simulink library "halin"  (R2021b)
settings: Solver=VariableStepAuto  StartTime=0.0  StopTime=10.0  RelTol=1e-3
undefined symbols (not defined in the file): KHAL_CAN1ABM1E2E_flg, KHAL_CAN1EPB1E2E_flg, KHAL_CAN1EPS1E2E_flg, KHAL_CAN1ESC1E2E_flg, KHAL_CAN1ESC5E2E_flg, KHAL_CAN3BMS1E2E_flg, KHAL_CAN3BMS6E2E_flg, KHAL_CAN3CCU1E2E_flg, KHAL_CAN3CCU2E2E_flg, KHAL_CAN3MCUNF1E2E_flg, KHAL_CAN3MCUNR1E2E_flg, KHAL_CAN3Shifter1E2E_flg, KHAL_CAN3Shifter2E2E_flg, KHAL_CAN6FCM2E2E_flg, KHAL_CAN6FCM4E2E_flg, TRUE
libraries: simulink x645, FVT_lib x207, hcu_lib x59
(part 16 of 23)

== system halin/HAL_IN/CAN4/zGW_LINFr2 ==
  DT_CAN4_SG_zGW_LINFr2 : Inport
  EWP1BlockError : Subsystem
  EWP1OverCurrError : Subsystem
  EWP2BlockError : Subsystem
  EWP2OverCurrError : Subsystem
  EWP3BlockError : Subsystem
  EWP3OverCurrError : Subsystem
  bus_selector : BusSelector  OutputSignals=CAN4_EWP1_Block_Error
  bus_selector1 : BusSelector  OutputSignals=CAN4_EWP1_OverCurr_Error
  bus_selector2 : BusSelector  OutputSignals=CAN4_EWP2_Block_Error
  bus_selector3 : BusSelector  OutputSignals=CAN4_EWP2_OverCurr_Error
  bus_selector4 : BusSelector  OutputSignals=CAN4_EWP3_Block_Error
  bus_selector5 : BusSelector  OutputSignals=CAN4_EWP3_OverCurr_Error
  VHAL_EWP1BlockError_enum : Outport
  VHAL_EWP1OverCurrError_enum : Outport  Port=2
  VHAL_EWP2BlockError_enum : Outport  Port=3
  VHAL_EWP2OverCurrError_enum : Outport  Port=4
  VHAL_EWP3BlockError_enum : Outport  Port=5
  VHAL_EWP3OverCurrError_enum : Outport  Port=6
  wires:
  DT_CAN4_SG_zGW_LINFr2/1 -> [DT_CAN4_SG_zGW_LINFr2]
  [DT_CAN4_SG_zGW_LINFr2] -> bus_selector/1
  bus_selector/1 -> EWP1BlockError/1(EWP1_Block_Error)  "<CAN4_EWP1_Block_Error>"
  EWP1BlockError/1(VHAL_EWP1BlockError_enum) -> VHAL_EWP1BlockError_enum/1
  [DT_CAN4_SG_zGW_LINFr2] -> bus_selector1/1
  bus_selector1/1 -> EWP1OverCurrError/1(EWP1_OverCurr_Error)  "<CAN4_EWP1_OverCurr_Error>"
  EWP1OverCurrError/1(VHAL_EWP1OverCurrError_enum) -> VHAL_EWP1OverCurrError_enum/1
  [DT_CAN4_SG_zGW_LINFr2] -> bus_selector2/1
  bus_selector2/1 -> EWP2BlockError/1(EWP2_Block_Error)  "<CAN4_EWP2_Block_Error>"
  EWP2BlockError/1(VHAL_EWP2BlockError_enum) -> VHAL_EWP2BlockError_enum/1
  [DT_CAN4_SG_zGW_LINFr2] -> bus_selector3/1
  bus_selector3/1 -> EWP2OverCurrError/1(EWP2_OverCurr_Error)  "<CAN4_EWP2_OverCurr_Error>"
  EWP2OverCurrError/1(VHAL_EWP2OverCurrError_enum) -> VHAL_EWP2OverCurrError_enum/1
  [DT_CAN4_SG_zGW_LINFr2] -> bus_selector4/1
  bus_selector4/1 -> EWP3BlockError/1(EWP3_Block_Error)  "<CAN4_EWP3_Block_Error>"
  EWP3BlockError/1(VHAL_EWP3BlockError_enum) -> VHAL_EWP3BlockError_enum/1
  [DT_CAN4_SG_zGW_LINFr2] -> bus_selector5/1
  bus_selector5/1 -> EWP3OverCurrError/1(EWP3_OverCurr_Error)  "<CAN4_EWP3_OverCurr_Error>"
  EWP3OverCurrError/1(VHAL_EWP3OverCurrError_enum) -> VHAL_EWP3OverCurrError_enum/1

== system halin/HAL_IN/CAN4/zGW_SEAT1 ==
  DT_CAN4_SG_zGW_SEAT1 : Inport
  DSEATAntiSta : Subsystem
  DSEATEntryFunSta : Subsystem
  DSEATErrorSta : Subsystem
  DSEATHWVer : Subsystem
  DSEATMode : Subsystem
  DSEATSWVer : Subsystem
  DSEATVentSta : Subsystem
  DSEATheatersta : Subsystem
  PSEATErrorSta : Subsystem
  PSEATHWVer : Subsystem
  PSEATMode : Subsystem
  PSEATSWVer : Subsystem
  PSEATVentSta : Subsystem
  PSEATheatersta : Subsystem
  bus_selector : BusSelector  OutputSignals=CAN4_DSEAT_Anti_Sta
  bus_selector1 : BusSelector  OutputSignals=CAN4_DSEAT_EntryFun_Sta
  bus_selector10 : BusSelector  OutputSignals=CAN4_PSEAT_Mode
  bus_selector11 : BusSelector  OutputSignals=CAN4_PSEAT_SW_Ver
  bus_selector12 : BusSelector  OutputSignals=CAN4_PSEAT_Vent_Sta
  bus_selector13 : BusSelector  OutputSignals=CAN4_PSEAT_heater_sta
  bus_selector2 : BusSelector  OutputSignals=CAN4_DSEAT_Error_Sta
  bus_selector3 : BusSelector  OutputSignals=CAN4_DSEAT_HW_Ver
  bus_selector4 : BusSelector  OutputSignals=CAN4_DSEAT_Mode
  bus_selector5 : BusSelector  OutputSignals=CAN4_DSEAT_SW_Ver
  bus_selector6 : BusSelector  OutputSignals=CAN4_DSEAT_Vent_Sta
  bus_selector7 : BusSelector  OutputSignals=CAN4_DSEAT_heater_sta
  bus_selector8 : BusSelector  OutputSignals=CAN4_PSEAT_Error_Sta
  bus_selector9 : BusSelector  OutputSignals=CAN4_PSEAT_HW_Ver
  VHAL_DSEATAntiSta_flg : Outport
  VHAL_DSEATEntryFunSta_flg : Outport  Port=2
  VHAL_DSEATErrorSta_flg : Outport  Port=3
  VHAL_DSEATHWVer_enum : Outport  Port=4
  VHAL_DSEATMode_enum : Outport  Port=5
  VHAL_DSEATSWVer_enum : Outport  Port=6
  VHAL_DSEATVentSta_enum : Outport  Port=7
  VHAL_DSEATheatersta_enum : Outport  Port=8
  VHAL_PSEATErrorSta_flg : Outport  Port=9
  VHAL_PSEATHWVer_enum : Outport  Port=10
  VHAL_PSEATMode_enum : Outport  Port=11
  VHAL_PSEATSWVer_enum : Outport  Port=12
  VHAL_PSEATVentSta_enum : Outport  Port=13
  VHAL_PSEATheatersta_enum : Outport  Port=14
  wires:
  DT_CAN4_SG_zGW_SEAT1/1 -> [DT_CAN4_SG_zGW_SEAT1]
  [DT_CAN4_SG_zGW_SEAT1] -> bus_selector/1
  bus_selector/1 -> DSEATAntiSta/1(DSEAT_Anti_Sta)  "<CAN4_DSEAT_Anti_Sta>"
  DSEATAntiSta/1(VHAL_DSEATAntiSta_flg) -> VHAL_DSEATAntiSta_flg/1
  [DT_CAN4_SG_zGW_SEAT1] -> bus_selector1/1
  bus_selector1/1 -> DSEATEntryFunSta/1(DSEAT_EntryFun_Sta)  "<CAN4_DSEAT_EntryFun_Sta>"
  DSEATEntryFunSta/1(VHAL_DSEATEntryFunSta_flg) -> VHAL_DSEATEntryFunSta_flg/1
  [DT_CAN4_SG_zGW_SEAT1] -> bus_selector2/1
  bus_selector2/1 -> DSEATErrorSta/1(DSEAT_Error_Sta)  "<CAN4_DSEAT_Error_Sta>"
  DSEATErrorSta/1(VHAL_DSEATErrorSta_flg) -> VHAL_DSEATErrorSta_flg/1
  [DT_CAN4_SG_zGW_SEAT1] -> bus_selector3/1
  bus_selector3/1 -> DSEATHWVer/1(DSEAT_HW_Ver)  "<CAN4_DSEAT_HW_Ver>"
  DSEATHWVer/1(VHAL_DSEATHWVer_enum) -> VHAL_DSEATHWVer_enum/1
  [DT_CAN4_SG_zGW_SEAT1] -> bus_selector4/1
  bus_selector4/1 -> DSEATMode/1(DSEAT_Mode)  "<CAN4_DSEAT_Mode>"
  DSEATMode/1(VHAL_DSEATMode_enum) -> VHAL_DSEATMode_enum/1
  [DT_CAN4_SG_zGW_SEAT1] -> bus_selector5/1
  bus_selector5/1 -> DSEATSWVer/1(DSEAT_SW_Ver)  "<CAN4_DSEAT_SW_Ver>"
  DSEATSWVer/1(VHAL_DSEATSWVer_enum) -> VHAL_DSEATSWVer_enum/1
  [DT_CAN4_SG_zGW_SEAT1] -> bus_selector6/1
  bus_selector6/1 -> DSEATVentSta/1(DSEAT_Vent_Sta)  "<CAN4_DSEAT_Vent_Sta>"
  DSEATVentSta/1(VHAL_DSEATVentSta_enum) -> VHAL_DSEATVentSta_enum/1
  [DT_CAN4_SG_zGW_SEAT1] -> bus_selector7/1
  bus_selector7/1 -> DSEATheatersta/1(DSEAT_heater_sta)  "<CAN4_DSEAT_heater_sta>"
  DSEATheatersta/1(VHAL_DSEATheatersta_enum) -> VHAL_DSEATheatersta_enum/1
  [DT_CAN4_SG_zGW_SEAT1] -> bus_selector8/1
  bus_selector8/1 -> PSEATErrorSta/1(PSEAT_Error_Sta)  "<CAN4_PSEAT_Error_Sta>"
  PSEATErrorSta/1(VHAL_PSEATErrorSta_flg) -> VHAL_PSEATErrorSta_flg/1
  [DT_CAN4_SG_zGW_SEAT1] -> bus_selector9/1
  bus_selector9/1 -> PSEATHWVer/1(PSEAT_HW_Ver)  "<CAN4_PSEAT_HW_Ver>"
  PSEATHWVer/1(VHAL_PSEATHWVer_enum) -> VHAL_PSEATHWVer_enum/1
  [DT_CAN4_SG_zGW_SEAT1] -> bus_selector10/1
  bus_selector10/1 -> PSEATMode/1(PSEAT_Mode)  "<CAN4_PSEAT_Mode>"
  PSEATMode/1(VHAL_PSEATMode_enum) -> VHAL_PSEATMode_enum/1
  [DT_CAN4_SG_zGW_SEAT1] -> bus_selector11/1
  bus_selector11/1 -> PSEATSWVer/1(PSEAT_SW_Ver)  "<CAN4_PSEAT_SW_Ver>"
  PSEATSWVer/1(VHAL_PSEATSWVer_enum) -> VHAL_PSEATSWVer_enum/1
  [DT_CAN4_SG_zGW_SEAT1] -> bus_selector12/1
  bus_selector12/1 -> PSEATVentSta/1(PSEAT_Vent_Sta)  "<CAN4_PSEAT_Vent_Sta>"
  PSEATVentSta/1(VHAL_PSEATVentSta_enum) -> VHAL_PSEATVentSta_enum/1
  [DT_CAN4_SG_zGW_SEAT1] -> bus_selector13/1
  bus_selector13/1 -> PSEATheatersta/1(PSEAT_heater_sta)  "<CAN4_PSEAT_heater_sta>"
  PSEATheatersta/1(VHAL_PSEATheatersta_enum) -> VHAL_PSEATheatersta_enum/1

== system halin/HAL_IN/CAN5/VHAL_CANMsgInvalidTBOX1_flg ==
  Cast To Boolean13 : DataTypeConversion  OutDataTypeStr=boolean
  Constant : Constant  Value=TRUE
  Latch13 : hcu_lib/Basic_Blocks/Latch
  Switch13 : Switch  Criteria=u2 ~= 0
  Unit Delay : UnitDelay  SampleTime=-1  HasFrameUpgradeWarning=on
  UnitConverter : DataTypeConversion  OutDataTypeStr=boolean
  Out : Outport
  wires:
  Constant/1 -> Switch13/3
  Unit Delay/1 -> Cast To Boolean13/1
  Cast To Boolean13/1 -> Switch13/1, Latch13/1
  Switch13/1 -> UnitConverter/1
  Latch13/1 -> Switch13/2
  UnitConverter/1 -> Unit Delay/1, Out/1  "VHAL_CANMsgInvalidTBOX1_flg"

== system halin/HAL_IN/CAN5/VHAL_CANMsgInvalidTBOX2_flg ==
  Cast To Boolean13 : DataTypeConversion  OutDataTypeStr=boolean
  Constant : Constant  Value=TRUE
  Latch13 : hcu_lib/Basic_Blocks/Latch
  Switch13 : Switch  Criteria=u2 ~= 0
  Unit Delay : UnitDelay  SampleTime=-1  HasFrameUpgradeWarning=on
  UnitConverter : DataTypeConversion  OutDataTypeStr=boolean
  Out : Outport
  wires:
  Constant/1 -> Switch13/3
  Unit Delay/1 -> Cast To Boolean13/1
  Cast To Boolean13/1 -> Switch13/1, Latch13/1
  Switch13/1 -> UnitConverter/1
  Latch13/1 -> Switch13/2
  UnitConverter/1 -> Unit Delay/1, Out/1  "VHAL_CANMsgInvalidTBOX2_flg"

== system halin/HAL_IN/CAN5/VHAL_CANMsgInvalidTBOX3_flg ==
  Cast To Boolean13 : DataTypeConversion  OutDataTypeStr=boolean
  Constant : Constant  Value=TRUE
  Latch13 : hcu_lib/Basic_Blocks/Latch
  Switch13 : Switch  Criteria=u2 ~= 0
  Unit Delay : UnitDelay  SampleTime=-1  HasFrameUpgradeWarning=on
  UnitConverter : DataTypeConversion  OutDataTypeStr=boolean
  Out : Outport
  wires:
  Constant/1 -> Switch13/3
  Unit Delay/1 -> Cast To Boolean13/1
  Cast To Boolean13/1 -> Switch13/1, Latch13/1
  Switch13/1 -> UnitConverter/1
  Latch13/1 -> Switch13/2
  UnitConverter/1 -> Unit Delay/1, Out/1  "VHAL_CANMsgInvalidTBOX3_flg"

== system halin/HAL_IN/CAN6/FCM1 ==
  DT_CAN6_SG_FCM1 : Inport
  ACCComfortBandLower : Subsystem
  ACCComfortBandUpper : Subsystem
  ACCJerkLowerLimit : Subsystem
  ACCJerkUpperLimit : Subsystem
  ACCObjDist : Subsystem
  ACCObjDstLvl : Subsystem
  ACCObjRelSpd : Subsystem
  ACCRequiredAccel : Subsystem
  ACCTakeoverReq : Subsystem
  ACCVehHoldReq : Subsystem
  ADASACCSta : Subsystem
  ADASAEBReq : Subsystem
  ADASAEBSta : Subsystem
  ADASCAMSpdLim : Subsystem
  ADASDBSReq : Subsystem
  ADASFCWMute : Subsystem
  ADASFCWSta : Subsystem
  ADASFaultSta : Subsystem
  ADASFltWrnReq : Subsystem
  ADASForceIdle : Subsystem
  ADASISASta : Subsystem
  ADASLDWMute : Subsystem
  ADASLDWSta : Subsystem
  ADASLFCHandsOffWarning : Subsystem
  ADASLFCSta : Subsystem
  ADASLFCWarnSound : Subsystem
  ADASLKASta : Subsystem
  ADASLaneModeL : Subsystem
  ADASLaneModeR : Subsystem
  ADASLanecurveL : Subsystem
  ADASLanecurveR : Subsystem
  ADASLanetypeL : Subsystem
  ADASLanetypeR : Subsystem
  ADASSLIFSpdLim : Subsystem
  ADASSLIFSta : Subsystem
  ADASShftPosnReq : Subsystem
  ADASShftPosnReqA : Subsystem
  ADASVehSpdLim : Subsystem
  ADASWarningMsg : Subsystem
  AEBVehHoldReq : Subsystem
  CameraBlockage : Subsystem
  FCM1Checksum : Subsystem
  FCM1LifeCount : Subsystem
  FCMACCmode : Subsystem
  FCMLKAStrToqReq : Subsystem
  FCMLKATOIAct : Subsystem
  FCMLKATOIFault : Subsystem
  ForceLowBeam : Subsystem
  HazardWarningReq : Subsystem
  ISAWarningMsg : Subsystem
  LKAHODDisplayWarning : Subsystem
  LKAHODSoundWarning : Subsystem
  LVDAACCStatusInformation : Subsystem
  LVDADisabled : Subsystem
  LVDAFailinfo : Subsystem
  LVDAMuteSta : Subsystem
  LVDAWarning : Subsystem
  LeftTurnLightReq : Subsystem
  RightTurnLightReq : Subsystem
  TargetType : Subsystem
  TimeGapLevel : Subsystem
  bus_selector : BusSelector  OutputSignals=CAN6_ACC_ComfortBandLower
  bus_selector1 : BusSelector  OutputSignals=CAN6_ACC_ComfortBandUpper
  bus_selector10 : BusSelector  OutputSignals=CAN6_ADAS_ACC_Sta
  bus_selector11 : BusSelector  OutputSignals=CAN6_ADAS_AEBReq
  bus_selector12 : BusSelector  OutputSignals=CAN6_ADAS_AEB_Sta
  bus_selector13 : BusSelector  OutputSignals=CAN6_ADAS_CAM_SpdLim
  bus_selector14 : BusSelector  OutputSignals=CAN6_ADAS_DBSReq
  bus_selector15 : BusSelector  OutputSignals=CAN6_ADAS_FCW_Mute
  bus_selector16 : BusSelector  OutputSignals=CAN6_ADAS_FCW_Sta
  bus_selector17 : BusSelector  OutputSignals=CAN6_ADAS_FaultSta
  bus_selector18 : BusSelector  OutputSignals=CAN6_ADAS_FltWrnReq
  bus_selector19 : BusSelector  OutputSignals=CAN6_ADAS_ForceIdle
  bus_selector2 : BusSelector  OutputSignals=CAN6_ACC_JerkLowerLimit
  bus_selector20 : BusSelector  OutputSignals=CAN6_ADAS_ISA_Sta
  bus_selector21 : BusSelector  OutputSignals=CAN6_ADAS_LDW_Mute
  bus_selector22 : BusSelector  OutputSignals=CAN6_ADAS_LDW_Sta
  bus_selector23 : BusSelector  OutputSignals=CAN6_ADAS_LFC_Hands_Off_Warning
  bus_selector24 : BusSelector  OutputSignals=CAN6_ADAS_LFC_Sta
  bus_selector25 : BusSelector  OutputSignals=CAN6_ADAS_LFC_Warn_Sound
  bus_selector26 : BusSelector  OutputSignals=CAN6_ADAS_LKA_Sta
  bus_selector27 : BusSelector  OutputSignals=CAN6_ADAS_LaneModeL
  bus_selector28 : BusSelector  OutputSignals=CAN6_ADAS_LaneModeR
  bus_selector29 : BusSelector  OutputSignals=CAN6_ADAS_Lane_curveL
  bus_selector3 : BusSelector  OutputSignals=CAN6_ACC_JerkUpperLimit
  bus_selector30 : BusSelector  OutputSignals=CAN6_ADAS_Lane_curveR
  bus_selector31 : BusSelector  OutputSignals=CAN6_ADAS_LanetypeL
  bus_selector32 : BusSelector  OutputSignals=CAN6_ADAS_LanetypeR
  bus_selector33 : BusSelector  OutputSignals=CAN6_ADAS_SLIF_SpdLim
  bus_selector34 : BusSelector  OutputSignals=CAN6_ADAS_SLIF_Sta
  bus_selector35 : BusSelector  OutputSignals=CAN6_ADAS_ShftPosnReq
  bus_selector36 : BusSelector  OutputSignals=CAN6_ADAS_ShftPosnReq_A
  bus_selector37 : BusSelector  OutputSignals=CAN6_ADAS_VehSpdLim
  bus_selector38 : BusSelector  OutputSignals=CAN6_ADAS_WarningMsg
  bus_selector39 : BusSelector  OutputSignals=CAN6_AEB_VehHoldReq
  bus_selector4 : BusSelector  OutputSignals=CAN6_ACC_ObjDist
  bus_selector40 : BusSelector  OutputSignals=CAN6_CameraBlockage
  bus_selector41 : BusSelector  OutputSignals=CAN6_FCM1_Checksum
  bus_selector42 : BusSelector  OutputSignals=CAN6_FCM1_LifeCount
  bus_selector43 : BusSelector  OutputSignals=CAN6_FCM_ACCmode
  bus_selector44 : BusSelector  OutputSignals=CAN6_FCM_LKA_StrToqReq
  bus_selector45 : BusSelector  OutputSignals=CAN6_FCM_LKA_TOIAct
  bus_selector46 : BusSelector  OutputSignals=CAN6_FCM_LKA_TOIFault
  bus_selector47 : BusSelector  OutputSignals=CAN6_ForceLowBeam
  bus_selector48 : BusSelector  OutputSignals=CAN6_HazardWarningReq
  bus_selector49 : BusSelector  OutputSignals=CAN6_ISA_WarningMsg
  bus_selector5 : BusSelector  OutputSignals=CAN6_ACC_ObjDstLvl
  bus_selector50 : BusSelector  OutputSignals=CAN6_LKA_HOD_Display_Warning
  bus_selector51 : BusSelector  OutputSignals=CAN6_LKA_HOD_Sound_Warning
  bus_selector52 : BusSelector  OutputSignals=CAN6_LVDA_ACCStatusInformation
  bus_selector53 : BusSelector  OutputSignals=CAN6_LVDA_Disabled
  bus_selector54 : BusSelector  OutputSignals=CAN6_LVDA_Failinfo
  bus_selector55 : BusSelector  OutputSignals=CAN6_LVDA_Mute_Sta
  bus_selector56 : BusSelector  OutputSignals=CAN6_LVDA_Warning
  bus_selector57 : BusSelector  OutputSignals=CAN6_LeftTurnLightReq
  bus_selector58 : BusSelector  OutputSignals=CAN6_RightTurnLightReq
  bus_selector59 : BusSelector  OutputSignals=CAN6_Target_Type
  bus_selector6 : BusSelector  OutputSignals=CAN6_ACC_ObjRelSpd
  bus_selector60 : BusSelector  OutputSignals=CAN6_TimeGapLevel
  bus_selector7 : BusSelector  OutputSignals=CAN6_ACC_RequiredAccel
  bus_selector8 : BusSelector  OutputSignals=CAN6_ACC_TakeoverReq
  bus_selector9 : BusSelector  OutputSignals=CAN6_ACC_VehHoldReq
  VHAL_ACCComfortBandLower_mps2 : Outport
  VHAL_ACCComfortBandUpper_mps2 : Outport  Port=2
  VHAL_ACCJerkLowerLimit_mps3 : Outport  Port=3
  VHAL_ACCJerkUpperLimit_mps3 : Outport  Port=4
  VHAL_ACCObjDist_m : Outport  Port=5
  VHAL_ACCObjDstLvl_enum : Outport  Port=6
  VHAL_ACCObjRelSpd_mps : Outport  Port=7
  VHAL_ACCRequiredAccel_mps2 : Outport  Port=8
  VHAL_ACCTakeoverReq_flg : Outport  Port=9
  VHAL_ACCVehHoldReq_flg : Outport  Port=10
  VHAL_ADASACCSta_enum : Outport  Port=11
  VHAL_ADASAEBReq_enum : Outport  Port=12
  VHAL_ADASAEBSta_enum : Outport  Port=13
  VHAL_ADASCAMSpdLim_enum : Outport  Port=14
  VHAL_ADASDBSReq_enum : Outport  Port=15
  VHAL_ADASFCWMute_flg : Outport  Port=16
  VHAL_ADASFCWSta_enum : Outport  Port=17
  VHAL_ADASFaultSta_flg : Outport  Port=18
  VHAL_ADASFltWrnReq_flg : Outport  Port=19
  VHAL_ADASForceIdle_flg : Outport  Port=20
  VHAL_ADASISASta_enum : Outport  Port=21
  VHAL_ADASLDWMute_flg : Outport  Port=22
  VHAL_ADASLDWSta_enum : Outport  Port=23
  VHAL_ADASLFCHandsOffWarning_enum : Outport  Port=24
  VHAL_ADASLFCSta_enum : Outport  Port=25
  VHAL_ADASLFCWarnSound_enum : Outport  Port=26
  VHAL_ADASLKASta_enum : Outport  Port=27
  VHAL_ADASLaneModeL_enum : Outport  Port=28
  VHAL_ADASLaneModeR_enum : Outport  Port=29
  VHAL_ADASLanecurveL_raw32 : Outport  Port=30
  VHAL_ADASLanecurveR_raw32 : Outport  Port=31
  VHAL_ADASLanetypeL_enum : Outport  Port=32
  VHAL_ADASLanetypeR_enum : Outport  Port=33
  VHAL_ADASSLIFSpdLim_enum : Outport  Port=34
  VHAL_ADASSLIFSta_enum : Outport  Port=35
  VHAL_ADASShftPosnReq_enum : Outport  Port=36
  VHAL_ADASShftPosnReqA_flg : Outport  Port=37
  VHAL_ADASVehSpdLim_enum : Outport  Port=38
  VHAL_ADASWarningMsg_enum : Outport  Port=39
  VHAL_AEBVehHoldReq_flg : Outport  Port=40
  VHAL_CameraBlockage_flg : Outport  Port=41
  VHAL_FCM1Checksum_enum : Outport  Port=42
  VHAL_FCM1LifeCount_enum : Outport  Port=43
  VHAL_FCMACCmode_enum : Outport  Port=44
  VHAL_FCMLKAStrToqReq_Nm : Outport  Port=45
  VHAL_FCMLKATOIAct_enum : Outport  Port=46
  VHAL_FCMLKATOIFault_flg : Outport  Port=47
  VHAL_ForceLowBeam_enum : Outport  Port=48
  VHAL_HazardWarningReq_flg : Outport  Port=49
  VHAL_ISAWarningMsg_enum : Outport  Port=50
  VHAL_LKAHODDisplayWarning_flg : Outport  Port=51
  VHAL_LKAHODSoundWarning_flg : Outport  Port=52
  VHAL_LVDAACCStatusInformation_flg : Outport  Port=53
  VHAL_LVDADisabled_flg : Outport  Port=54
  VHAL_LVDAFailinfo_flg : Outport  Port=55
  VHAL_LVDAMuteSta_enum : Outport  Port=56
  VHAL_LVDAWarning_flg : Outport  Port=57
  VHAL_LeftTurnLightReq_flg : Outport  Port=58
  VHAL_RightTurnLightReq_flg : Outport  Port=59
  VHAL_TargetType_enum : Outport  Port=60
  VHAL_TimeGapLevel_enum : Outport  Port=61
  wires:
  DT_CAN6_SG_FCM1/1 -> [DT_CAN6_SG_FCM1]
  [DT_CAN6_SG_FCM1] -> bus_selector/1
  bus_selector/1 -> ACCComfortBandLower/1(ACC_ComfortBandLower)  "<CAN6_ACC_ComfortBandLower>"
  ACCComfortBandLower/1(VHAL_ACCComfortBandLower_mps2) -> VHAL_ACCComfortBandLower_mps2/1
  [DT_CAN6_SG_FCM1] -> bus_selector1/1
  bus_selector1/1 -> ACCComfortBandUpper/1(ACC_ComfortBandUpper)  "<CAN6_ACC_ComfortBandUpper>"
  ACCComfortBandUpper/1(VHAL_ACCComfortBandUpper_mps2) -> VHAL_ACCComfortBandUpper_mps2/1
  [DT_CAN6_SG_FCM1] -> bus_selector2/1
  bus_selector2/1 -> ACCJerkLowerLimit/1(ACC_JerkLowerLimit)  "<CAN6_ACC_JerkLowerLimit>"
  ACCJerkLowerLimit/1(VHAL_ACCJerkLowerLimit_mps3) -> VHAL_ACCJerkLowerLimit_mps3/1
  [DT_CAN6_SG_FCM1] -> bus_selector3/1
  bus_selector3/1 -> ACCJerkUpperLimit/1(ACC_JerkUpperLimit)  "<CAN6_ACC_JerkUpperLimit>"
  ACCJerkUpperLimit/1(VHAL_ACCJerkUpperLimit_mps3) -> VHAL_ACCJerkUpperLimit_mps3/1
  [DT_CAN6_SG_FCM1] -> bus_selector4/1
  bus_selector4/1 -> ACCObjDist/1(ACC_ObjDist)  "<CAN6_ACC_ObjDist>"
  ACCObjDist/1(VHAL_ACCObjDist_m) -> VHAL_ACCObjDist_m/1
  [DT_CAN6_SG_FCM1] -> bus_selector5/1
  bus_selector5/1 -> ACCObjDstLvl/1(ACC_ObjDstLvl)  "<CAN6_ACC_ObjDstLvl>"
  ACCObjDstLvl/1(VHAL_ACCObjDstLvl_enum) -> VHAL_ACCObjDstLvl_enum/1
  [DT_CAN6_SG_FCM1] -> bus_selector6/1
  bus_selector6/1 -> ACCObjRelSpd/1(ACC_ObjRelSpd)  "<CAN6_ACC_ObjRelSpd>"
  ACCObjRelSpd/1(VHAL_ACCObjRelSpd_mps) -> VHAL_ACCObjRelSpd_mps/1
  [DT_CAN6_SG_FCM1] -> bus_selector7/1
  bus_selector7/1 -> ACCRequiredAccel/1(ACC_RequiredAccel)  "<CAN6_ACC_RequiredAccel>"
  ACCRequiredAccel/1(VHAL_ACCRequiredAccel_mps2) -> VHAL_ACCRequiredAccel_mps2/1
  [DT_CAN6_SG_FCM1] -> bus_selector8/1
  bus_selector8/1 -> ACCTakeoverReq/1(ACC_TakeoverReq)  "<CAN6_ACC_TakeoverReq>"
  ACCTakeoverReq/1(VHAL_ACCTakeoverReq_flg) -> VHAL_ACCTakeoverReq_flg/1
  [DT_CAN6_SG_FCM1] -> bus_selector9/1
  bus_selector9/1 -> ACCVehHoldReq/1(ACC_VehHoldReq)  "<CAN6_ACC_VehHoldReq>"
  ACCVehHoldReq/1(VHAL_ACCVehHoldReq_flg) -> VHAL_ACCVehHoldReq_flg/1
  [DT_CAN6_SG_FCM1] -> bus_selector10/1
  bus_selector10/1 -> ADASACCSta/1(ADAS_ACC_Sta)  "<CAN6_ADAS_ACC_Sta>"
  ADASACCSta/1(VHAL_ADASACCSta_enum) -> VHAL_ADASACCSta_enum/1
  [DT_CAN6_SG_FCM1] -> bus_selector11/1
  bus_selector11/1 -> ADASAEBReq/1(ADAS_AEBReq)  "<CAN6_ADAS_AEBReq>"
  ADASAEBReq/1(VHAL_ADASAEBReq_enum) -> VHAL_ADASAEBReq_enum/1
  [DT_CAN6_SG_FCM1] -> bus_selector12/1
  bus_selector12/1 -> ADASAEBSta/1(ADAS_AEB_Sta)  "<CAN6_ADAS_AEB_Sta>"
  ADASAEBSta/1(VHAL_ADASAEBSta_enum) -> VHAL_ADASAEBSta_enum/1
  [DT_CAN6_SG_FCM1] -> bus_selector13/1
  bus_selector13/1 -> ADASCAMSpdLim/1(ADAS_CAM_SpdLim)  "<CAN6_ADAS_CAM_SpdLim>"
  ADASCAMSpdLim/1(VHAL_ADASCAMSpdLim_enum) -> VHAL_ADASCAMSpdLim_enum/1
  [DT_CAN6_SG_FCM1] -> bus_selector14/1
  bus_selector14/1 -> ADASDBSReq/1(ADAS_DBSReq)  "<CAN6_ADAS_DBSReq>"
  ADASDBSReq/1(VHAL_ADASDBSReq_enum) -> VHAL_ADASDBSReq_enum/1
  [DT_CAN6_SG_FCM1] -> bus_selector15/1
  bus_selector15/1 -> ADASFCWMute/1(ADAS_FCW_Mute)  "<CAN6_ADAS_FCW_Mute>"
  ADASFCWMute/1(VHAL_ADASFCWMute_flg) -> VHAL_ADASFCWMute_flg/1
  [DT_CAN6_SG_FCM1] -> bus_selector16/1
  bus_selector16/1 -> ADASFCWSta/1(ADAS_FCW_Sta)  "<CAN6_ADAS_FCW_Sta>"
  ADASFCWSta/1(VHAL_ADASFCWSta_enum) -> VHAL_ADASFCWSta_enum/1
  [DT_CAN6_SG_FCM1] -> bus_selector17/1
  bus_selector17/1 -> ADASFaultSta/1(ADAS_FaultSta)  "<CAN6_ADAS_FaultSta>"
  ADASFaultSta/1(VHAL_ADASFaultSta_flg) -> VHAL_ADASFaultSta_flg/1
  [DT_CAN6_SG_FCM1] -> bus_selector18/1
  bus_selector18/1 -> ADASFltWrnReq/1(ADAS_FltWrnReq)  "<CAN6_ADAS_FltWrnReq>"
  ADASFltWrnReq/1(VHAL_ADASFltWrnReq_flg) -> VHAL_ADASFltWrnReq_flg/1
  [DT_CAN6_SG_FCM1] -> bus_selector19/1
  bus_selector19/1 -> ADASForceIdle/1(ADAS_ForceIdle)  "<CAN6_ADAS_ForceIdle>"
  ADASForceIdle/1(VHAL_ADASForceIdle_flg) -> VHAL_ADASForceIdle_flg/1
  [DT_CAN6_SG_FCM1] -> bus_selector20/1
  bus_selector20/1 -> ADASISASta/1(ADAS_ISA_Sta)  "<CAN6_ADAS_ISA_Sta>"
  ADASISASta/1(VHAL_ADASISASta_enum) -> VHAL_ADASISASta_enum/1
  [DT_CAN6_SG_FCM1] -> bus_selector21/1
  bus_selector21/1 -> ADASLDWMute/1(ADAS_LDW_Mute)  "<CAN6_ADAS_LDW_Mute>"
  ADASLDWMute/1(VHAL_ADASLDWMute_flg) -> VHAL_ADASLDWMute_flg/1
  [DT_CAN6_SG_FCM1] -> bus_selector22/1
  bus_selector22/1 -> ADASLDWSta/1(ADAS_LDW_Sta)  "<CAN6_ADAS_LDW_Sta>"
  ADASLDWSta/1(VHAL_ADASLDWSta_enum) -> VHAL_ADASLDWSta_enum/1
  [DT_CAN6_SG_FCM1] -> bus_selector23/1
  bus_selector23/1 -> ADASLFCHandsOffWarning/1(ADAS_LFC_Hands_Off_Warning)  "<CAN6_ADAS_LFC_Hands_Off_Warning>"
  ADASLFCHandsOffWarning/1(VHAL_ADASLFCHandsOffWarning_enum) -> VHAL_ADASLFCHandsOffWarning_enum/1
  [DT_CAN6_SG_FCM1] -> bus_selector24/1
  bus_selector24/1 -> ADASLFCSta/1(ADAS_LFC_Sta)  "<CAN6_ADAS_LFC_Sta>"
  ADASLFCSta/1(VHAL_ADASLFCSta_enum) -> VHAL_ADASLFCSta_enum/1
  [DT_CAN6_SG_FCM1] -> bus_selector25/1
  bus_selector25/1 -> ADASLFCWarnSound/1(ADAS_LFC_Warn_Sound)  "<CAN6_ADAS_LFC_Warn_Sound>"
  ADASLFCWarnSound/1(VHAL_ADASLFCWarnSound_enum) -> VHAL_ADASLFCWarnSound_enum/1
  [DT_CAN6_SG_FCM1] -> bus_selector26/1
  bus_selector26/1 -> ADASLKASta/1(ADAS_LKA_Sta)  "<CAN6_ADAS_LKA_Sta>"
  ADASLKASta/1(VHAL_ADASLKASta_enum) -> VHAL_ADASLKASta_enum/1
  [DT_CAN6_SG_FCM1] -> bus_selector27/1
  bus_selector27/1 -> ADASLaneModeL/1(ADAS_LaneModeL)  "<CAN6_ADAS_LaneModeL>"
  ADASLaneModeL/1(VHAL_ADASLaneModeL_enum) -> VHAL_ADASLaneModeL_enum/1
  [DT_CAN6_SG_FCM1] -> bus_selector28/1
  bus_selector28/1 -> ADASLaneModeR/1(ADAS_LaneModeR)  "<CAN6_ADAS_LaneModeR>"
  ADASLaneModeR/1(VHAL_ADASLaneModeR_enum) -> VHAL_ADASLaneModeR_enum/1
  [DT_CAN6_SG_FCM1] -> bus_selector29/1
  bus_selector29/1 -> ADASLanecurveL/1(ADAS_Lane_curveL)  "<CAN6_ADAS_Lane_curveL>"
  ADASLanecurveL/1(VHAL_ADASLanecurveL_raw32) -> VHAL_ADASLanecurveL_raw32/1
  [DT_CAN6_SG_FCM1] -> bus_selector30/1
  bus_selector30/1 -> ADASLanecurveR/1(ADAS_Lane_curveR)  "<CAN6_ADAS_Lane_curveR>"
  ADASLanecurveR/1(VHAL_ADASLanecurveR_raw32) -> VHAL_ADASLanecurveR_raw32/1
  [DT_CAN6_SG_FCM1] -> bus_selector31/1
  bus_selector31/1 -> ADASLanetypeL/1(ADAS_LanetypeL)  "<CAN6_ADAS_LanetypeL>"
  ADASLanetypeL/1(VHAL_ADASLanetypeL_enum) -> VHAL_ADASLanetypeL_enum/1
  [DT_CAN6_SG_FCM1] -> bus_selector32/1
  bus_selector32/1 -> ADASLanetypeR/1(ADAS_LanetypeR)  "<CAN6_ADAS_LanetypeR>"
  ADASLanetypeR/1(VHAL_ADASLanetypeR_enum) -> VHAL_ADASLanetypeR_enum/1
  [DT_CAN6_SG_FCM1] -> bus_selector33/1
  bus_selector33/1 -> ADASSLIFSpdLim/1(ADAS_SLIF_SpdLim)  "<CAN6_ADAS_SLIF_SpdLim>"
  ADASSLIFSpdLim/1(VHAL_ADASSLIFSpdLim_enum) -> VHAL_ADASSLIFSpdLim_enum/1
  [DT_CAN6_SG_FCM1] -> bus_selector34/1
  bus_selector34/1 -> ADASSLIFSta/1(ADAS_SLIF_Sta)  "<CAN6_ADAS_SLIF_Sta>"
  ADASSLIFSta/1(VHAL_ADASSLIFSta_enum) -> VHAL_ADASSLIFSta_enum/1
  [DT_CAN6_SG_FCM1] -> bus_selector35/1
  bus_selector35/1 -> ADASShftPosnReq/1(ADAS_ShftPosnReq)  "<CAN6_ADAS_ShftPosnReq>"
  ADASShftPosnReq/1(VHAL_ADASShftPosnReq_enum) -> VHAL_ADASShftPosnReq_enum/1
  [DT_CAN6_SG_FCM1] -> bus_selector36/1
  bus_selector36/1 -> ADASShftPosnReqA/1(ADAS_ShftPosnReq_A)  "<CAN6_ADAS_ShftPosnReq_A>"
  ADASShftPosnReqA/1(VHAL_ADASShftPosnReqA_flg) -> VHAL_ADASShftPosnReqA_flg/1
  [DT_CAN6_SG_FCM1] -> bus_selector37/1
  bus_selector37/1 -> ADASVehSpdLim/1(ADAS_VehSpdLim)  "<CAN6_ADAS_VehSpdLim>"
  ADASVehSpdLim/1(VHAL_ADASVehSpdLim_enum) -> VHAL_ADASVehSpdLim_enum/1
  [DT_CAN6_SG_FCM1] -> bus_selector38/1
  bus_selector38/1 -> ADASWarningMsg/1(ADAS_WarningMsg)  "<CAN6_ADAS_WarningMsg>"
  ADASWarningMsg/1(VHAL_ADASWarningMsg_enum) -> VHAL_ADASWarningMsg_enum/1
  [DT_CAN6_SG_FCM1] -> bus_selector39/1
  bus_selector39/1 -> AEBVehHoldReq/1(AEB_VehHoldReq)  "<CAN6_AEB_VehHoldReq>"
  AEBVehHoldReq/1(VHAL_AEBVehHoldReq_flg) -> VHAL_AEBVehHoldReq_flg/1
  [DT_CAN6_SG_FCM1] -> bus_selector40/1
  bus_selector40/1 -> CameraBlockage/1(CameraBlockage)  "<CAN6_CameraBlockage>"
  CameraBlockage/1(VHAL_CameraBlockage_flg) -> VHAL_CameraBlockage_flg/1
  [DT_CAN6_SG_FCM1] -> bus_selector41/1
  bus_selector41/1 -> FCM1Checksum/1(FCM1_Checksum)  "<CAN6_FCM1_Checksum>"
  FCM1Checksum/1(VHAL_FCM1Checksum_enum) -> VHAL_FCM1Checksum_enum/1
  [DT_CAN6_SG_FCM1] -> bus_selector42/1
  bus_selector42/1 -> FCM1LifeCount/1(FCM1_LifeCount)  "<CAN6_FCM1_LifeCount>"
  FCM1LifeCount/1(VHAL_FCM1LifeCount_enum) -> VHAL_FCM1LifeCount_enum/1
  [DT_CAN6_SG_FCM1] -> bus_selector43/1
  bus_selector43/1 -> FCMACCmode/1(FCM_ACCmode)  "<CAN6_FCM_ACCmode>"
  FCMACCmode/1(VHAL_FCMACCmode_enum) -> VHAL_FCMACCmode_enum/1
  [DT_CAN6_SG_FCM1] -> bus_selector44/1
  bus_selector44/1 -> FCMLKAStrToqReq/1(FCM_LKA_StrToqReq)  "<CAN6_FCM_LKA_StrToqReq>"
  FCMLKAStrToqReq/1(VHAL_FCMLKAStrToqReq_Nm) -> VHAL_FCMLKAStrToqReq_Nm/1
  [DT_CAN6_SG_FCM1] -> bus_selector45/1
  bus_selector45/1 -> FCMLKATOIAct/1(FCM_LKA_TOIAct)  "<CAN6_FCM_LKA_TOIAct>"
  FCMLKATOIAct/1(VHAL_FCMLKATOIAct_enum) -> VHAL_FCMLKATOIAct_enum/1
  [DT_CAN6_SG_FCM1] -> bus_selector46/1
  bus_selector46/1 -> FCMLKATOIFault/1(FCM_LKA_TOIFault)  "<CAN6_FCM_LKA_TOIFault>"
  FCMLKATOIFault/1(VHAL_FCMLKATOIFault_flg) -> VHAL_FCMLKATOIFault_flg/1
  [DT_CAN6_SG_FCM1] -> bus_selector47/1
  bus_selector47/1 -> ForceLowBeam/1(ForceLowBeam)  "<CAN6_ForceLowBeam>"
  ForceLowBeam/1(VHAL_ForceLowBeam_enum) -> VHAL_ForceLowBeam_enum/1
  [DT_CAN6_SG_FCM1] -> bus_selector48/1
  bus_selector48/1 -> HazardWarningReq/1(HazardWarningReq)  "<CAN6_HazardWarningReq>"
  HazardWarningReq/1(VHAL_HazardWarningReq_flg) -> VHAL_HazardWarningReq_flg/1
  [DT_CAN6_SG_FCM1] -> bus_selector49/1
  bus_selector49/1 -> ISAWarningMsg/1(ISA_WarningMsg)  "<CAN6_ISA_WarningMsg>"
  ISAWarningMsg/1(VHAL_ISAWarningMsg_enum) -> VHAL_ISAWarningMsg_enum/1
  [DT_CAN6_SG_FCM1] -> bus_selector50/1
  bus_selector50/1 -> LKAHODDisplayWarning/1(LKA_HOD_Display_Warning)  "<CAN6_LKA_HOD_Display_Warning>"
  LKAHODDisplayWarning/1(VHAL_LKAHODDisplayWarning_flg) -> VHAL_LKAHODDisplayWarning_flg/1
  [DT_CAN6_SG_FCM1] -> bus_selector51/1
  bus_selector51/1 -> LKAHODSoundWarning/1(LKA_HOD_Sound_Warning)  "<CAN6_LKA_HOD_Sound_Warning>"
  LKAHODSoundWarning/1(VHAL_LKAHODSoundWarning_flg) -> VHAL_LKAHODSoundWarning_flg/1
  [DT_CAN6_SG_FCM1] -> bus_selector52/1
  bus_selector52/1 -> LVDAACCStatusInformation/1(LVDA_ACCStatusInformation)  "<CAN6_LVDA_ACCStatusInformation>"
  LVDAACCStatusInformation/1(VHAL_LVDAACCStatusInformation_flg) -> VHAL_LVDAACCStatusInformation_flg/1
  [DT_CAN6_SG_FCM1] -> bus_selector53/1
  bus_selector53/1 -> LVDADisabled/1(LVDA_Disabled)  "<CAN6_LVDA_Disabled>"
  LVDADisabled/1(VHAL_LVDADisabled_flg) -> VHAL_LVDADisabled_flg/1
  [DT_CAN6_SG_FCM1] -> bus_selector54/1
  bus_selector54/1 -> LVDAFailinfo/1(LVDA_Failinfo)  "<CAN6_LVDA_Failinfo>"
  LVDAFailinfo/1(VHAL_LVDAFailinfo_flg) -> VHAL_LVDAFailinfo_flg/1
  [DT_CAN6_SG_FCM1] -> bus_selector55/1
  bus_selector55/1 -> LVDAMuteSta/1(LVDA_Mute_Sta)  "<CAN6_LVDA_Mute_Sta>"
  LVDAMuteSta/1(VHAL_LVDAMuteSta_enum) -> VHAL_LVDAMuteSta_enum/1
  [DT_CAN6_SG_FCM1] -> bus_selector56/1
  bus_selector56/1 -> LVDAWarning/1(LVDA_Warning)  "<CAN6_LVDA_Warning>"
  LVDAWarning/1(VHAL_LVDAWarning_flg) -> VHAL_LVDAWarning_flg/1
  [DT_CAN6_SG_FCM1] -> bus_selector57/1
  bus_selector57/1 -> LeftTurnLightReq/1(LeftTurnLightReq)  "<CAN6_LeftTurnLightReq>"
  LeftTurnLightReq/1(VHAL_LeftTurnLightReq_flg) -> VHAL_LeftTurnLightReq_flg/1
  [DT_CAN6_SG_FCM1] -> bus_selector58/1
  bus_selector58/1 -> RightTurnLightReq/1(RightTurnLightReq)  "<CAN6_RightTurnLightReq>"
  RightTurnLightReq/1(VHAL_RightTurnLightReq_flg) -> VHAL_RightTurnLightReq_flg/1
  [DT_CAN6_SG_FCM1] -> bus_selector59/1
  bus_selector59/1 -> TargetType/1(Target_Type)  "<CAN6_Target_Type>"
  TargetType/1(VHAL_TargetType_enum) -> VHAL_TargetType_enum/1
  [DT_CAN6_SG_FCM1] -> bus_selector60/1
  bus_selector60/1 -> TimeGapLevel/1(TimeGapLevel)  "<CAN6_TimeGapLevel>"
  TimeGapLevel/1(VHAL_TimeGapLevel_enum) -> VHAL_TimeGapLevel_enum/1
